simulink model "motorcondelay"  (R2017a)
settings: Solver=VariableStepAuto  StartTime=0.0  StopTime=10  RelTol=1e-3
values from neighbouring files (symbols this model uses):
  k = 0.97287    [Region_de_estabilidad.m]
  ki = 51.39    [Region_de_estabilidad.m]
  kp = 4.266    [Region_de_estabilidad.m]
  m = 1    [Region_de_estabilidad.m]
  ts = 0.02    [Region_de_estabilidad.m]
settings Model: Creator=MarioAndres  LastModifiedBy=MarioAndres

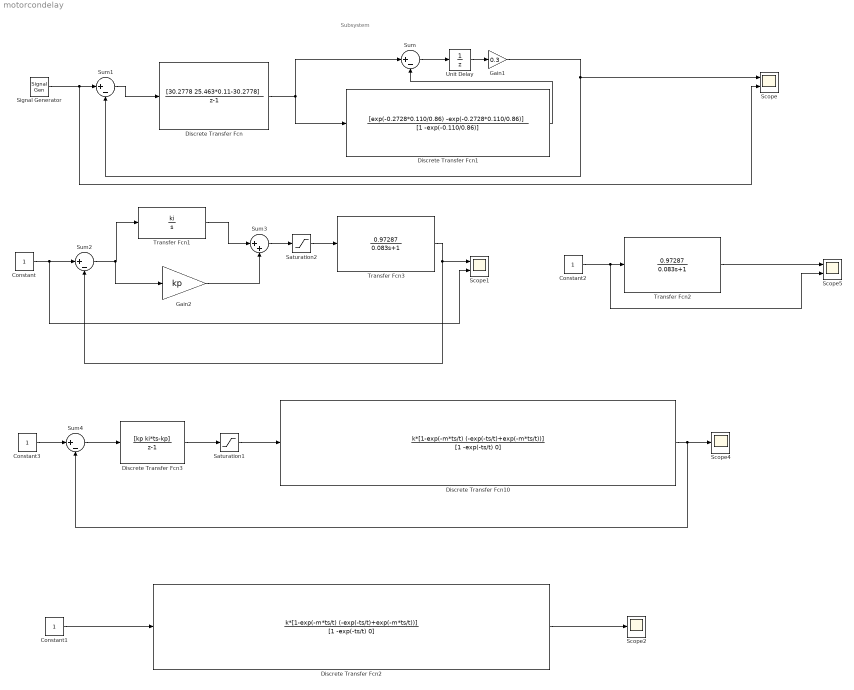
== system motorcondelay ==
  note: Subsystem
  Constant{,1..3} (4 alike) : Constant
  Discrete Transfer Fcn : DiscreteTransferFcn  Numerator=[30.2778 25.463*0.11-30.2778]  Denominator=[1 -1]  SampleTime=0.11
  Discrete Transfer Fcn1 : DiscreteTransferFcn  Numerator=[exp(-0.2728*0.110/0.86) -exp(-0.2728*0.110/0.86)]  Denominator=[1 -exp(-0.110/0.86)]  SampleTime=0.11
  Discrete Transfer Fcn10 : DiscreteTransferFcn  Numerator=k*[1-exp(-m*ts/t) (-exp(-ts/t)+exp(-m*ts/t))]  Denominator=[1 -exp(-ts/t) 0]  SampleTime=ts
  Discrete Transfer Fcn2 : DiscreteTransferFcn  Numerator=k*[1-exp(-m*ts/t) (-exp(-ts/t)+exp(-m*ts/t))]  Denominator=[1 -exp(-ts/t) 0]  SampleTime=ts
  Discrete Transfer Fcn3 : DiscreteTransferFcn  Numerator=[kp ki*ts-kp]  Denominator=[1 -1]  SampleTime=ts
  Gain1 : Gain  Gain=0.3
  Gain2 : Gain  Gain=kp
  Saturation1 : Saturate  UpperLimit=2.75  LowerLimit=0.55  LinearizeAsGain=off
  Saturation2 : Saturate  UpperLimit=2.25  LowerLimit=0.55  LinearizeAsGain=off
  Scope : Scope  NumInputPorts=2
  Scope1 : Scope  NumInputPorts=2
  Scope2 : Scope
  Scope4 : Scope
  Scope5 : Scope  NumInputPorts=2
  Signal Generator : SignalGenerator  WaveForm=square  Frequency=1/5
  Sum{,1..2,4} (4 alike) : Sum  Inputs=|+-
  Sum3 : Sum  Inputs=|++
  Transfer Fcn1 : TransferFcn  Numerator=ki  Denominator=[1 0]
  Transfer Fcn2 : TransferFcn  Numerator=[0.97287]  Denominator=[0.083 1]
  Transfer Fcn3 : TransferFcn  Numerator=[0.97287]  Denominator=[0.083 1]
  Unit Delay : UnitDelay  SampleTime=0.11
  wires:
  Signal Generator/1 -> Scope/2, Sum1/1
  Sum1/1 -> Discrete Transfer Fcn/1
  Gain1/1 -> Sum1/2, Scope/1
  Unit Delay/1 -> Gain1/1
  Discrete Transfer Fcn/1 -> Discrete Transfer Fcn1/1, Sum/1
  Sum/1 -> Unit Delay/1
  Discrete Transfer Fcn1/1 -> Sum/2
  Transfer Fcn3/1 -> Sum2/2, Scope1/1
  Sum2/1 -> Gain2/1, Transfer Fcn1/1
  Constant/1 -> Scope1/2, Sum2/1
  Transfer Fcn2/1 -> Scope5/1
  Constant2/1 -> Scope5/2, Transfer Fcn2/1
  Sum4/1 -> Discrete Transfer Fcn3/1
  Constant3/1 -> Sum4/1
  Discrete Transfer Fcn10/1 -> Scope4/1, Sum4/2
  Discrete Transfer Fcn3/1 -> Saturation1/1
  Transfer Fcn1/1 -> Sum3/1
  Gain2/1 -> Sum3/2
  Sum3/1 -> Saturation2/1
  Saturation1/1 -> Discrete Transfer Fcn10/1
  Saturation2/1 -> Transfer Fcn3/1
  Constant1/1 -> Discrete Transfer Fcn2/1
  Discrete Transfer Fcn2/1 -> Scope2/1
